simulink model "Rudder_system_control2022"  (R2022b)
settings: Solver=VariableStepAuto  StartTime=0.0  StopTime=10.0  RelTol=1e-3
values from neighbouring files (symbols this model uses):
  Fg = 1    [start.m]
  H = 1    [start.m]
  Js = 1    [start.m]
settings Model: Creator=victo  LastModifiedBy=matheusassis
settings SolverCC: AlgebraicLoopSolver=TrustRegion
settings DebuggingCC: UnconnectedInputMsg=warning  UnconnectedOutputMsg=warning  UnconnectedLineMsg=warning  SFMachineParentedDataDiag=warning
settings ModelReferenceCC: EnableRefExpFcnMdlSchedulingChecks=on

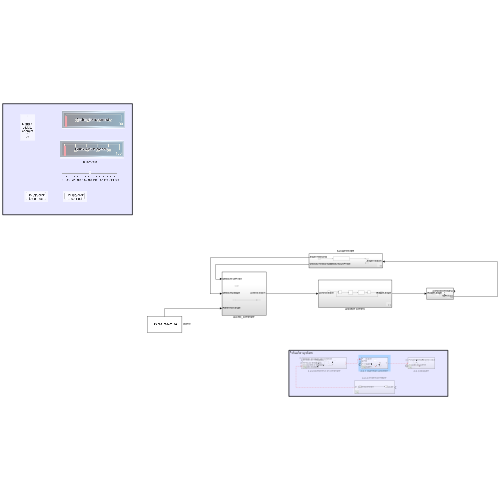
[thumbnail: Simulink's stored preview of the top-level diagram]
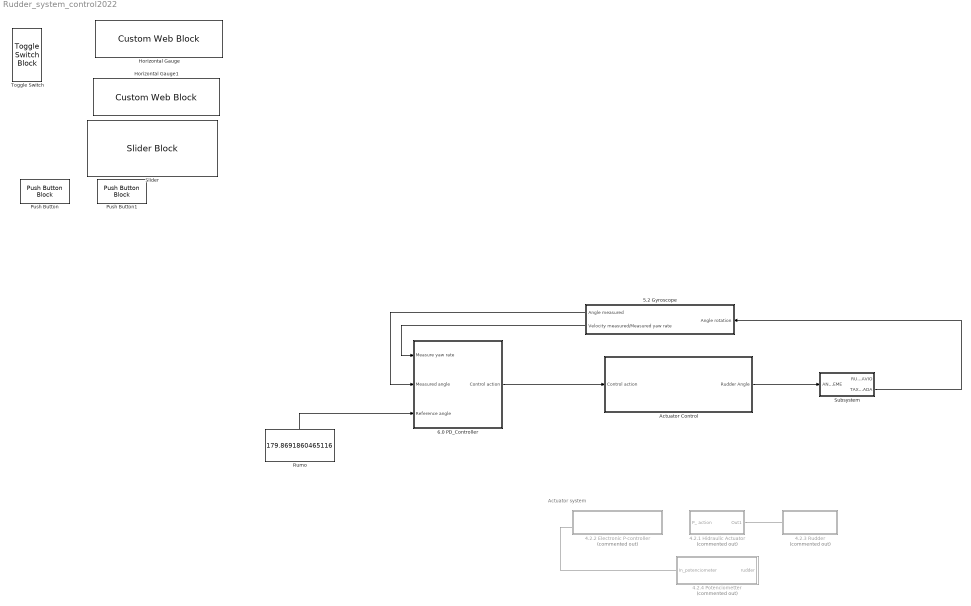
== system Rudder_system_control2022 ==
  note: Actuator system
  4.2.1 Hidraulic Actuator : Subsystem  Commented=on
  4.2.2 Electronic P-controller : Subsystem  Commented=on
  4.2.3 Rudder : Subsystem  Commented=on
  4.2.4 Potenciometter : Subsystem  Commented=on
  5.2 Gyroscope : Subsystem
  6.0 PD_Controller : Subsystem
  Actuator Control : Subsystem
  Horizontal Gauge : CustomWebBlock  ShowInitialText=on  Configuration="{\"type\":\"LinearGauge\",\"settings\":{\"BindingType\":\"signal\",\"fixedAspectRatio\":\"on\",\"orientation\":\"horizontal\"},\"components\":[{\"name\":\"LinearScaleComponent\",\"settings\":{\"bounds\":{\"max\":100,\"min\":0,\"tickInterval\":\"auto\"},\"labelColor\":[250,245,199],\"labelFont\":{\"font\":\"Arial\",\"fontSize\":12},\"labelOffset\":0.05,\"labelTransparency\":1,\"needleImage\":{\"size\":[21,75],\"src\":\"data:image/svg+xml;base64,PHN2ZyB4bWxucz0iaHR0cDovL3d3dy53My5vcmcvMjAwMC9zdmciIHhtbG5zOnhsaW5rPSJodHRwOi8vd3d3LnczLm9yZy8xOTk5L3hsaW5rIiB2aWV3Qm94PSIwIDAgMjEgNzUiPjxkZWZzPjxzdHlsZT4uY2xzLTF7ZmlsbDpub25lO30uY2xzLTJ7aXNvbGF0aW9uOmlzb2xhdGU7fS5jbHMtM3tjbGlwLXBhdGg6dXJsKCNjbGlwLXBhdGgpO30uY2xzLTR7b3BhY2l0eTowLjM7bWl4LWJsZW5kLW1vZGU6bXVsdGlwbHk7fS5jbHMtNXtmaWxsOiNlYjI2Mjk7fTwvc3R5bGU+PGNsaXBQYXRoIGlkPSJjbGlwLXBhdGgiIHRyYW5zZm9y ...(+1928 chars)\",\"srcOrientation\":\"Right\"},\"needleOffset\":[0,0.01094391244870041],\"needleSize\":{\"height\":0.7589285714285714,\"width\":0.11960078534031414},\"position\":[0.06986607142857143,0.01995798319327731,0.9641544117647058,0.8],\"referencePoint\":\"auto\",\"scaleColorSize\":0.24,\"scaleColors\":[],\"scaleColorsSize\":0.2,\"scaleDirection\":\"LR\",\"tickColor\":[250,245,200],\"tickTransparency\":1,\"valueBarColor\":[23,89,176],\"valueBarSize\":0.23,\"valueBarTransparency\":1}},{\"name\":\"BackgroundImageComponent\",\"settings\":{\"image\":{\"size\":[380,101],\"src\":\"data:image/svg+xml;base64,PHN2ZyB4bWxucz0iaHR0cDovL3d3dy53My5vcmcvMjAwMC9zdmciIHhtbG5zOnhsaW5rPSJodHRwOi8vd3d3LnczLm9yZy8xOTk5L3hsaW5rIiB2aWV3Qm94PSIwIDAgMzgwIDEwMSI+PGRlZnM+PHN0eWxlPi5jbHMtMXtmaWxsOnVybCgjbGluZWFyLWdyYWRpZW50KTt9LmNscy0ye2ZpbGw6dXJsKCNsaW5lYXItZ3JhZGllbnQtMik7fS5jbHMtM3tmaWxsOnVybCgjbGluZWFyLWdyYWRpZW50LTMpO308L3N0eWxlPjxsaW5lYXJHcmFkaWVudCBpZD0ibGluZWFyLWdyYWRpZW50IiB5MT0iNTAuNSIgeDI9IjM5OS4yOCIgeTI9IjUw ...(+2216 chars)\",\"srcOrientation\":\"horizontal\"},\"position\":[0,0,1,1],\"scaleMode\":\"0\"}}]}"
  Horizontal Gauge1 : CustomWebBlock  ShowInitialText=on  Configuration="{\"type\":\"LinearGauge\",\"settings\":{\"BindingType\":\"signal\",\"fixedAspectRatio\":\"on\",\"orientation\":\"horizontal\"},\"components\":[{\"name\":\"LinearScaleComponent\",\"settings\":{\"bounds\":{\"max\":100,\"min\":0,\"tickInterval\":\"auto\"},\"labelColor\":[250,245,199],\"labelFont\":{\"font\":\"Arial\",\"fontSize\":12},\"labelOffset\":0.05,\"labelTransparency\":1,\"needleImage\":{\"size\":[21,75],\"src\":\"data:image/svg+xml;base64,PHN2ZyB4bWxucz0iaHR0cDovL3d3dy53My5vcmcvMjAwMC9zdmciIHhtbG5zOnhsaW5rPSJodHRwOi8vd3d3LnczLm9yZy8xOTk5L3hsaW5rIiB2aWV3Qm94PSIwIDAgMjEgNzUiPjxkZWZzPjxzdHlsZT4uY2xzLTF7ZmlsbDpub25lO30uY2xzLTJ7aXNvbGF0aW9uOmlzb2xhdGU7fS5jbHMtM3tjbGlwLXBhdGg6dXJsKCNjbGlwLXBhdGgpO30uY2xzLTR7b3BhY2l0eTowLjM7bWl4LWJsZW5kLW1vZGU6bXVsdGlwbHk7fS5jbHMtNXtmaWxsOiNlYjI2Mjk7fTwvc3R5bGU+PGNsaXBQYXRoIGlkPSJjbGlwLXBhdGgiIHRyYW5zZm9y ...(+1928 chars)\",\"srcOrientation\":\"Right\"},\"needleOffset\":[0,0.01094391244870041],\"needleSize\":{\"height\":0.7589285714285714,\"width\":0.11960078534031414},\"position\":[0.06986607142857143,0.01995798319327731,0.9641544117647058,0.8],\"referencePoint\":\"auto\",\"scaleColorSize\":0.24,\"scaleColors\":[],\"scaleColorsSize\":0.2,\"scaleDirection\":\"LR\",\"tickColor\":[250,245,200],\"tickTransparency\":1,\"valueBarColor\":[23,89,176],\"valueBarSize\":0.23,\"valueBarTransparency\":1}},{\"name\":\"BackgroundImageComponent\",\"settings\":{\"image\":{\"size\":[380,101],\"src\":\"data:image/svg+xml;base64,PHN2ZyB4bWxucz0iaHR0cDovL3d3dy53My5vcmcvMjAwMC9zdmciIHhtbG5zOnhsaW5rPSJodHRwOi8vd3d3LnczLm9yZy8xOTk5L3hsaW5rIiB2aWV3Qm94PSIwIDAgMzgwIDEwMSI+PGRlZnM+PHN0eWxlPi5jbHMtMXtmaWxsOnVybCgjbGluZWFyLWdyYWRpZW50KTt9LmNscy0ye2ZpbGw6dXJsKCNsaW5lYXItZ3JhZGllbnQtMik7fS5jbHMtM3tmaWxsOnVybCgjbGluZWFyLWdyYWRpZW50LTMpO308L3N0eWxlPjxsaW5lYXJHcmFkaWVudCBpZD0ibGluZWFyLWdyYWRpZW50IiB5MT0iNTAuNSIgeDI9IjM5OS4yOCIgeTI9IjUw ...(+2216 chars)\",\"srcOrientation\":\"horizontal\"},\"position\":[0,0,1,1],\"scaleMode\":\"0\"}}]}"
  Push Button : PushButtonBlock
  Push Button1 : PushButtonBlock
  Rumo : Constant  Value=179.8691860465116  VectorParams1D=off
  Slider : SliderBlock  ScaleMax=360
  Subsystem : Subsystem
  Toggle Switch : ToggleSwitchBlock
      settings: Values={{'Off', 'On'}, [0 1]}
  wires:
  5.2 Gyroscope/2(Velocity measured/Measured yaw rate) -> 6.0 PD_Controller/1(Measure yaw rate)
  5.2 Gyroscope/1(Angle measured) -> 6.0 PD_Controller/2(Measured angle)
  Subsystem/2(TAXA DE GUINADA) -> 5.2 Gyroscope/1(Angle rotation)
  4.2.1 Hidraulic Actuator/1(Out1) -> ?
  ? -> 4.2.1 Hidraulic Actuator/1(P_ action)
  4.2.4 Potenciometter/1(In_potenciometer) -> ?
  Rumo/1 -> 6.0 PD_Controller/3(Reference angle)
  6.0 PD_Controller/1(Control action) -> Actuator Control/1(Control action)
  Actuator Control/1(Rudder Angle) -> Subsystem/1(ANGULO DE LEME)

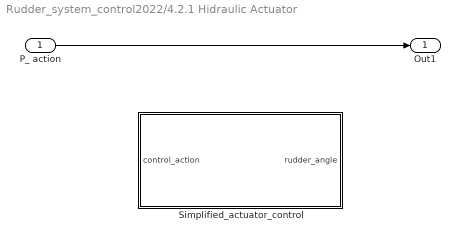
== system Rudder_system_control2022/4.2.1 Hidraulic Actuator ==
  P_ action : Inport
  Simplified_actuator_control : Subsystem
  Out1 : Outport
  wires:
  P_ action/1 -> Out1/1

== system Rudder_system_control2022/4.2.2 Electronic P-controller ==

== system Rudder_system_control2022/4.2.3 Rudder ==

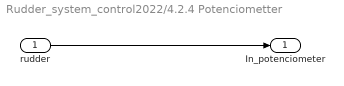
== system Rudder_system_control2022/4.2.4 Potenciometter ==
  rudder : Inport
  In_potenciometer : Outport
  wires:
  rudder/1 -> In_potenciometer/1

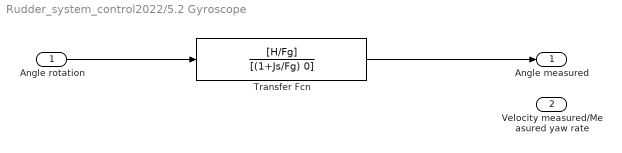
== system Rudder_system_control2022/5.2 Gyroscope ==
  Angle rotation : Inport
  Transfer Fcn : TransferFcn  Numerator=[H/Fg]  Denominator=[(1+Js/Fg) 0]
  Angle measured : Outport
  Velocity measured/Measured yaw rate : Outport  Port=2
  wires:
  Angle rotation/1 -> Transfer Fcn/1
  Transfer Fcn/1 -> Angle measured/1

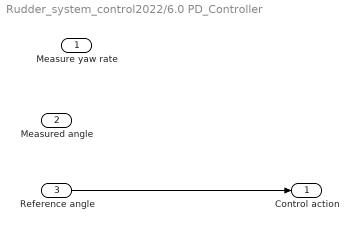
== system Rudder_system_control2022/6.0 PD_Controller ==
  Measure yaw rate : Inport
  Measured angle : Inport  Port=2
  Reference angle : Inport  Port=3
  Control action : Outport
  wires:
  Reference angle/1 -> Control action/1

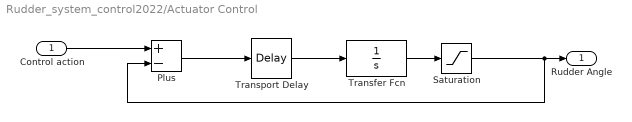
== system Rudder_system_control2022/Actuator Control ==
  Control action : Inport
  Plus : Sum  Inputs=+-
  Saturation : Saturate  UpperLimit=30  LowerLimit=-30
  Transfer Fcn : TransferFcn  Denominator=[1 0]
  Transport Delay : TransportDelay
  Rudder Angle : Outport
  wires:
  Saturation/1 -> Plus/2, Rudder Angle/1
  Plus/1 -> Transport Delay/1
  Control action/1 -> Plus/1
  Transport Delay/1 -> Transfer Fcn/1
  Transfer Fcn/1 -> Saturation/1

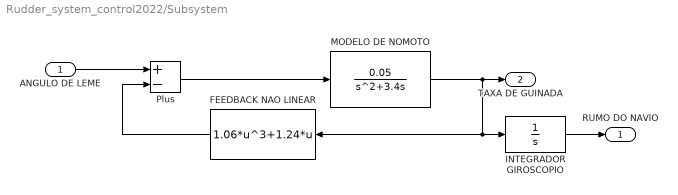
== system Rudder_system_control2022/Subsystem ==
  ANGULO DE LEME : Inport
  FEEDBACK NAO LINEAR : Fcn  Expr=1.06*u^3+1.24*u
  INTEGRADOR GIROSCOPIO : TransferFcn  Denominator=[1 0]
  MODELO DE NOMOTO : TransferFcn  Numerator=[0.05]  Denominator=[1 3.4 0]
  Plus : Sum  Inputs=+-
  RUMO DO NAVIO : Outport
  TAXA DE GUINADA : Outport  Port=2
  wires:
  INTEGRADOR GIROSCOPIO/1 -> RUMO DO NAVIO/1
  FEEDBACK NAO LINEAR/1 -> Plus/2
  ANGULO DE LEME/1 -> Plus/1
  MODELO DE NOMOTO/1 -> FEEDBACK NAO LINEAR/1, INTEGRADOR GIROSCOPIO/1, TAXA DE GUINADA/1
  Plus/1 -> MODELO DE NOMOTO/1

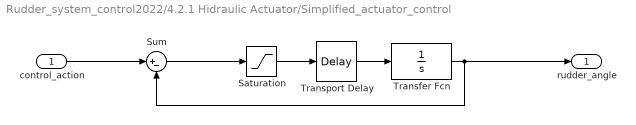
== system Rudder_system_control2022/4.2.1 Hidraulic Actuator/Simplified_actuator_control ==
  control_action : Inport
  Saturation : Saturate  UpperLimit=35  LowerLimit=35
  Sum : Sum  Inputs=|+-
  Transfer Fcn : TransferFcn  Denominator=[1 0]
  Transport Delay : TransportDelay
  rudder_angle : Outport
  wires:
  Transport Delay/1 -> Transfer Fcn/1
  control_action/1 -> Sum/1
  Sum/1 -> Saturation/1
  Saturation/1 -> Transport Delay/1
  Transfer Fcn/1 -> Sum/2, rudder_angle/1
